simulink model "my_model2"  (R2019b)
settings: Solver=VariableStepAuto  StartTime=0.0  StopTime=10.0  RelTol=1e-3
settings Model: Creator=admin  LastModifiedBy=admin
settings DataIOCC: ReturnWorkspaceOutputs=off

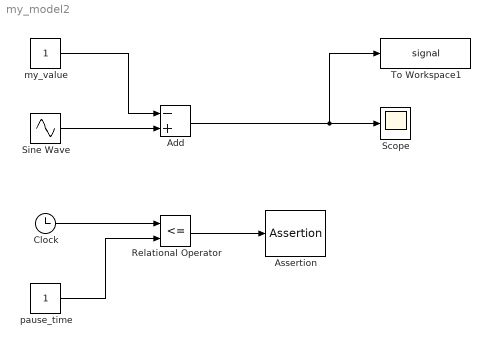
== system my_model2 ==
  Add : Sum  Inputs=-+
  Assertion : Assertion  AssertionFailFcn=set_param(bdroot, 'SimulationCommand', 'pause')  StopWhenAssertionFail=off
  Clock : Clock
  Relational Operator : RelationalOperator  Operator=<=  OutDataTypeStr=boolean  RndMeth=Simplest
  Scope : Scope
      settings: StartFcn=open_system(gcbh);
  Sine Wave : Sin  SampleTime=0
  To Workspace1 : ToWorkspace  VariableName=signal  SampleTime=0.1
  my_value : Constant
  pause_time : Constant
  wires:
  Add/1 -> To Workspace1/1, Scope/1
  Sine Wave/1 -> Add/2
  my_value/1 -> Add/1
  Clock/1 -> Relational Operator/1
  Relational Operator/1 -> Assertion/1
  pause_time/1 -> Relational Operator/2
